simulink model "Junctions7"  (Simulink 8.7)
settings: Solver=ode45  StartTime=0.0  StopTime=10.0  RelTol=1e-3
settings Model: Creator=scaife  LastModifiedBy=hamza  ExtModeAutoUpdateStatusClock=off
settings DataIOCC: SignalLoggingSaveFormat=ModelDataLogs  SignalLoggingName=sigsOut
settings DebuggingCC: SaveWithParameterizedLinksMsg=none  SignalResolutionControl=TryResolveAllWithWarning  MultiTaskDSMMsg=warning  MultiTaskCondExecSysMsg=none  StrictBusMsg=None
settings HardwareCC: TargetUnknown=on
settings SFSimCC: SimParseCustomCode=off
settings GRTTargetCC: GeneratePreprocessorConditionals=Use local settings  CombineOutputUpdateFcns=off  GRTInterface=on

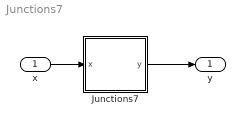
== system Junctions7 ==
  x : Inport
  Junctions7 : Stateflow chart  TreatAsAtomicUnit=on
  y : Outport
  wires:
  Junctions7/1(y) -> y/1
  x/1 -> Junctions7/1(x)

== stateflow chart Junctions7 ==
  state A
  state B
  A -> (junction 7) [order 1] : [x<>0]{y++}
  (junction 7) -> B : [x<2]
  (default) -> A
  A -> (junction 7) [order 2] : [x==0]{y--}
  data: x input int32; y output int32
